simulink model "TESTE_RAMPA"  (R2020a)
settings: Solver=VariableStepAuto  StartTime=0.0  StopTime=20.0  RelTol=1e-3
libraries: simulink x1
settings Model: Creator=jguil  LastModifiedBy=jguil

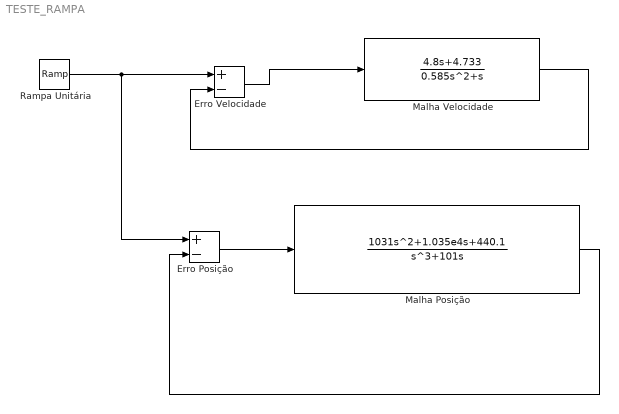
== system TESTE_RAMPA ==
  Erro Posição : Sum  Inputs=+-
  Erro Velocidade : Sum  Inputs=+-
  Malha Posição : TransferFcn  Numerator=[1031 1.035e4 440.1 ]  Denominator=[1 0 101 0]
  Malha Velocidade : TransferFcn  Numerator=[4.8 4.733]  Denominator=[0.585 1 0]
  Rampa Unitária : simulink/Sources/Ramp  slope=1  start=0  InitialOutput=0
  wires:
  Rampa Unitária/1 -> Erro Posição/1, Erro Velocidade/1
  Malha Velocidade/1 -> Erro Velocidade/2
  Erro Velocidade/1 -> Malha Velocidade/1
  Malha Posição/1 -> Erro Posição/2
  Erro Posição/1 -> Malha Posição/1
